simulink model "RCAM_Simulation"  (R2020a)
settings: Solver=VariableStepAuto  StartTime=0.0  StopTime=TF  RelTol=1e-3
InitFcn:
  | %Initialize constants for the RCAM simulation
  | clear; clc; close all
  | 
  | %% Define Constants
  | 
  | % Initially airplane going 165 knots at pitch of 5.73 degrees
  | x0 = [95;
  |       0;
  |       0;
  |       0;
  |       0;
  |       0;
  |       0;
  |       0.1;
  |       0];
  | 
  | x_ref = [100;
  |         0;
  |         0;
  |         0;
  |         0;
  |         0;
  |         0;
  |         0;
  |         0];
  | 
  | u = [0;
  |     -0.1;
  |     0;
  |     0.08;
  |     0.08];  % u2 initially at -5.73 degrees
  |                               % u4 and u5 at minimum initially
  | 
  | TF = 3*60;                      %sec, simulation time
  | 
  | % Saturation of Aileron Deflection, d_A
  | u1min = -25*pi/180;
  | u1max =  25*pi/180;
  | 
  | % Saturation of Tailplane (Horizontal Stabilizer) Deflection, d_T
  | u2min = -25*pi/180;
  | u2max =  10*pi/180;
  | 
  | % Saturation of Rudder Deflection, d_R
  | u3min = -30*pi/180;
  | u3max =  30*pi/180;
  | 
  | % Saturation of Throttle 1, d_TH1
  | u4min = 0.5*pi/180;
  | u4max =  10*pi/180;
  | 
  | % Saturation of Throttle 2, d_TH2
  | u5min = 0.5*pi/180;
  | u5max =  10*pi/180;
  | 
  | 
  | A_Linear = [-0.0446016164153414,0,0.0240349082743274,0,3.52183512710970,0,0,-9.80350406554132,0;
  | 0,-0.212333323695311,0,-3.64070000000000,0,-99.9337000000000,9.80350178873670,0,0;
  | -0.225748711836021,0,-0.818399711955672,0,96.6710635864611,0,0,0.357006987153097,0;
  | 0,-0.0335341188805878,0,-1.58352903033459,0,0.687344310697465,0,0,0;
  | -0.00295055240857513,0,-0.0389521422511313,0,-1.30090635747471,0,0,0,0;
  | 0,0.0108256600646234,0,0.0651934906310271,0,-0.650931103680959,0,0,0;
  | 0,0,0,1,0,-0.0364160847060240,0,0,0;
  | 0,0,0,0,1,0,0,0,0;
  | 0,0,0,0,0,1.00066284593029,0,0,0];
  | 
  | B_Linear = [0,-0.368697023171135,0,9.81000392264348,9.81000392264348;
  | 0,0,3.18499971085933,0,0;
  | 0,-10.1199839259439,0,0,0;
  | -1.31295051980772,0,0.503855989256257,0.0407489669716354,-0.0407489669716354;
  | 0,-4.03508162593975,0,0.392399973265370,0.392399973265370;
  | -0.0274928904316402,0,-0.564836211864184,0.780393997313998,-0.780393997313998;
  | 0,0,0,0,0;
  | 0,0,0,0,0;
  | 0,0,0,0,0];
  | 
  | [K_Linear,S_Linear,CLP] = lqr(A_Linear, B_Linear, eye(9), 0.1*eye(5));
StopFcn:
  | figure(1)
  | 
  | subplot(3,3,1)
  | plot(out.X.Time, out.X.Data(:,1))
  | title('velocity in x-axis')
  | xlabel('time, second')
  | ylabel('u, m/s')
  | 
  | subplot(3,3,2)
  | plot(out.X.Time, out.X.Data(:,2))
  | title('velocity in y-axis')
  | xlabel('time, second')
  | ylabel('v, m/s')
  | 
  | subplot(3,3,3)
  | plot(out.X.Time, out.X.Data(:,3))
  | title('velocity in z-axis')
  | xlabel('time, second')
  | ylabel('w, m/s')
  | 
  | subplot(3,3,4)
  | plot(out.X.Time, out.X.Data(:,4))
  | title('angular velocity about x-axis')
  | xlabel('time, second')
  | ylabel('p, rad/s')
  | 
  | subplot(3,3,5)
  | plot(out.X.Time, out.X.Data(:,5))
  | title('angular velocity about y-axis')
  | xlabel('time, second')
  | ylabel('q, rad/s')
  | 
  | subplot(3,3,6)
  | plot(out.X.Time, out.X.Data(:,6))
  | title('angular velocity about z-axis')
  | xlabel('time, second')
  | ylabel('r, rad/s')
  | 
  | subplot(3,3,7)
  | plot(out.X.Time, out.X.Data(:,7))
  | title('Roll Euler Angle')
  | xlabel('time, second')
  | ylabel('phi, rad')
  | 
  | subplot(3,3,8)
  | plot(out.X.Time, out.X.Data(:,8))
  | title('Pitch Euler Angle')
  | xlabel('time, second')
  | ylabel('theta, rad')
  | 
  | subplot(3,3,9)
  | plot(out.X.Time, out.X.Data(:,9))
  | title('Yaw Euler Angle')
  | xlabel('time, second')
  | ylabel('psi, rad')
  | 
  | Number = length(out.U.Time);
  | 
  | figure(2)
  | subplot(5,1,1)
  | plot(out.U.Time, out.U.Data(:,1))
  | title('Aileron Deflection')
  | xlabel('time, second')
  | ylabel('\delta_A, rad')
  | hold on
  | plot(out.U.Time, -25*pi/180*ones(Number),'r-')
  | plot(out.U.Time, 25*pi/180*ones(Number),'r-')
  | 
  | subplot(5,1,2)
  | plot(out.U.Time, out.U.Data(:,2))
  | title('Horizontal Stabilizer Deflection')
  | xlabel('time, second')
  | ylabel('\delta_S, rad')
  | hold on
  | plot(out.U.Time, -25*pi/180*ones(Number),'r-')
  | plot(out.U.Time, 10*pi/180*ones(Number),'r-')
  | 
  | subplot(5,1,3)
  | plot(out.U.Time, out.U.Data(:,3))
  | title('Rudder Deflection')
  | xlabel('time, second')
  | ylabel('\delta_R, rad')
  | hold on
  | plot(out.U.Time, -30*pi/180*ones(Number),'r-')
  | plot(out.U.Time, 30*pi/180*ones(Number),'r-')
  | 
  | subplot(5,1,4)
  | plot(out.U.Time, out.U.Data(:,4))
  | title('Throttle 1')
  | xlabel('time, second')
  | ylabel('\delta_th1, rad')
  | hold on
  | plot(out.U.Time, -0.5*pi/180*ones(Number),'r-')
  | plot(out.U.Time, 10*pi/180*ones(Number),'r-')
  | 
  | subplot(5,1,5)
  | plot(out.U.Time, out.U.Data(:,5))
  | title('Throttle 2')
  | xlabel('time, second')
  | ylabel('\delta_th2, rad')
  | hold on
  | plot(out.U.Time, -0.5*pi/180*ones(Number),'r-')
  | plot(out.U.Time, 10*pi/180*ones(Number),'r-')
values from neighbouring files (symbols this model uses):
  out = sim('RCAM_Simulation.slx')    [Starting_Simulation.m]
undefined symbols (not defined in the file or in its folder): K_Linear, RCAM_model
libraries: aerolibutil x2, vrlib x1
settings Model: Creator=Edward Han  LastModifiedBy=Edward Han

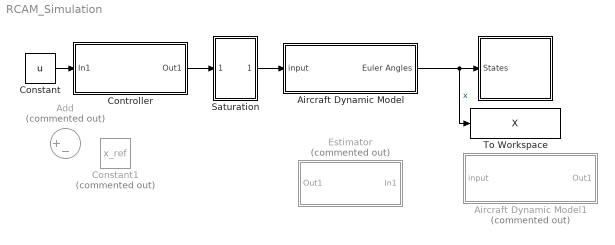
== system RCAM_Simulation ==
  " " : Subsystem
  Add : Sum  Commented=on  Inputs=|+-
  Aircraft Dynamic Model : Subsystem
  Aircraft Dynamic Model1 : Subsystem  Commented=on
  Constant : Constant  Value=u
  Constant1 : Constant  Commented=on  Value=x_ref
  Controller : Subsystem
  Estimator : Subsystem  Commented=on
  Saturation : Subsystem
  To Workspace : ToWorkspace  VariableName=X  SaveFormat=Timeseries  SampleTime=-1
  wires:
  Aircraft Dynamic Model/1(Euler Angles) -> " "/1(States), To Workspace/1  "x"
  Saturation/1(input) -> Aircraft Dynamic Model/1(input)
  Constant/1 -> Controller/1(In1)
  Controller/1(Out1) -> Saturation/1(In1)

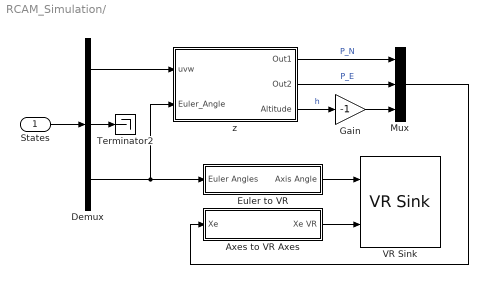
== system RCAM_Simulation/  ==
  States : Inport
  Axes to VR Axes : Subsystem
  Demux : Demux  Outputs=[3,3,3]
  Euler to VR : Subsystem
  Gain : Gain  Gain=-1
  Mux : Mux  Inputs=3
  Terminator2 : Terminator
  VR Sink : vrlib/VR Sink  InstantiateOnLoad=on  SampleTime=0.1  ViewEnable=on  RemoteChange=off  RemoteView=off  FieldsWritten=HL20.rotation.4.1.1.double#HL20.translation.3.1.1.double  WorldFileName=aeroblk_HL20.wrl  WorldDescription=aeroblk_HL20  AutoView=on  VideoDimensions=[]  AllowVariableSize=off
  z : Subsystem
  wires:
  Axes to VR Axes/1(Xe VR) -> VR Sink/2
  Euler to VR/1(Axis Angle) -> VR Sink/1
  Mux/1 -> Axes to VR Axes/1(Xe)
  States/1 -> Demux/1
  Demux/3 -> z/2(Euler_Angle), Euler to VR/1(Euler Angles)
  Demux/1 -> z/1(uvw)
  Demux/2 -> Terminator2/1
  z/3(Altitude) -> Gain/1  "h"
  z/1(Out1) -> Mux/1  "P_N"
  z/2(Out2) -> Mux/2  "P_E"
  Gain/1 -> Mux/3

== system RCAM_Simulation/Aircraft Dynamic Model ==
  input : Inport
  Integrator : Integrator  InitialCondition=x0
  Interpreted MATLAB Function : MATLABFcn  MATLABFcn=RCAM_model(u(1:9),u(10:14))
  Mux : Mux  Inputs=2
  To Workspace1 : ToWorkspace  VariableName=U  SaveFormat=Timeseries  SampleTime=-1
  Euler Angles : Outport
  wires:
  Integrator/1 -> Euler Angles/1, Mux/1
  Interpreted MATLAB Function/1 -> Integrator/1  "XDOT(9x1)"
  input/1 -> To Workspace1/1, Mux/2
  Mux/1 -> Interpreted MATLAB Function/1  "x_and_u"

== system RCAM_Simulation/Aircraft Dynamic Model1 ==
  input : Inport
  State-Space : StateSpace  A=A_Linear  B=B_Linear  C=eye(9)  D=zeros(9,5)  InitialCondition=x0
  To Workspace1 : ToWorkspace  VariableName=U  SaveFormat=Timeseries  SampleTime=-1
  Out1 : Outport
  wires:
  input/1 -> To Workspace1/1, State-Space/1
  State-Space/1 -> Out1/1

== system RCAM_Simulation/Controller ==
  In1 : Inport
  Gain : Gain  Commented=on  Gain=K_Linear  Multiplication=Matrix(K*u)
  PID : Subsystem  Commented=on
  Out1 : Outport
  wires:
  In1/1 -> Out1/1

== system RCAM_Simulation/Estimator ==
  In1 : Inport
  Out1 : Outport
  wires:
  In1/1 -> Out1/1

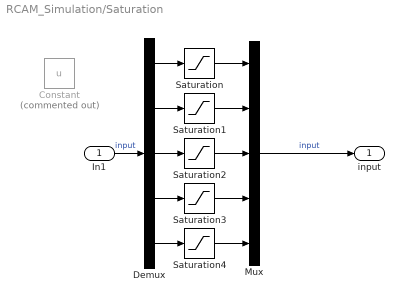
== system RCAM_Simulation/Saturation ==
  In1 : Inport
  Constant : Constant  Commented=on  Value=u
  Demux : Demux  Outputs=5
  Mux : Mux  Inputs=5
  Saturation : Saturate  UpperLimit=u1max  LowerLimit=u1min
  Saturation1 : Saturate  UpperLimit=u2max  LowerLimit=u2min
  Saturation2 : Saturate  UpperLimit=u3max  LowerLimit=u3min
  Saturation3 : Saturate  UpperLimit=u4max  LowerLimit=u4min
  Saturation4 : Saturate  UpperLimit=u5max  LowerLimit=u5min
  input : Outport
  wires:
  In1/1 -> Demux/1  "input"
  Saturation4/1 -> Mux/5
  Saturation3/1 -> Mux/4
  Demux/3 -> Saturation2/1
  Demux/1 -> Saturation/1
  Demux/2 -> Saturation1/1
  Saturation2/1 -> Mux/3
  Demux/4 -> Saturation3/1
  Demux/5 -> Saturation4/1
  Saturation/1 -> Mux/1
  Mux/1 -> input/1  "input"
  Saturation1/1 -> Mux/2

== system RCAM_Simulation/ /Axes to VR Axes ==
  Xe : Inport
  Concatenate : Concatenate  NumInputs=3
  Demux : Demux  Outputs=3
      settings: DisplayOption=none
  rad-->deg : Gain  Gain=-1  SaturateOnIntegerOverflow=on  OutDataTypeStr=Inherit: Same as input  ParamDataTypeStr=Inherit: Same as input
  rad-->deg1 : Gain  Gain=-1  SaturateOnIntegerOverflow=on  OutDataTypeStr=Inherit: Same as input  ParamDataTypeStr=Inherit: Same as input
  Xe VR : Outport  VectorParamsAs1DForOutWhenUnconnected=off
  wires:
  Xe/1 -> Demux/1
  Demux/1 -> Concatenate/1
  Demux/2 -> rad-->deg/1
  Demux/3 -> rad-->deg1/1
  Concatenate/1 -> Xe VR/1
  rad-->deg1/1 -> Concatenate/2
  rad-->deg/1 -> Concatenate/3

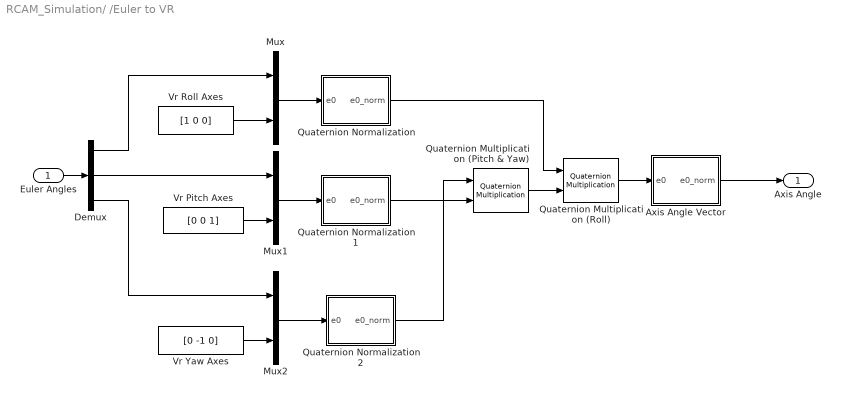
== system RCAM_Simulation/ /Euler to VR ==
  Euler Angles : Inport
  Axis Angle Vector : Subsystem
  Demux : Demux  Outputs=3
      settings: DisplayOption=none
  Mux : Mux  Inputs=2
  Mux1 : Mux  Inputs=2
  Mux2 : Mux  Inputs=2
  Quaternion Multiplication (Pitch & Yaw) : aerolibutil/Quaternion Multiplication
  Quaternion Multiplication (Roll) : aerolibutil/Quaternion Multiplication
  Quaternion Normalization : Subsystem
  Quaternion Normalization1 : Subsystem
  Quaternion Normalization2 : Subsystem
  Vr Pitch Axes : Constant  Value=[0 0 1]
  Vr Roll Axes : Constant  Value=[1 0 0]
  Vr Yaw Axes : Constant  Value=[0 -1 0]
  Axis Angle : Outport  VectorParamsAs1DForOutWhenUnconnected=off
  wires:
  Quaternion Multiplication (Roll)/1 -> Axis Angle Vector/1(e0)
  Quaternion Multiplication (Pitch & Yaw)/1 -> Quaternion Multiplication (Roll)/2
  Axis Angle Vector/1(e0_norm) -> Axis Angle/1
  Quaternion Normalization/1(e0_norm) -> Quaternion Multiplication (Roll)/1
  Quaternion Normalization2/1(e0_norm) -> Quaternion Multiplication (Pitch & Yaw)/1
  Quaternion Normalization1/1(e0_norm) -> Quaternion Multiplication (Pitch & Yaw)/2
  Mux2/1 -> Quaternion Normalization2/1(e0)
  Mux1/1 -> Quaternion Normalization1/1(e0)
  Mux/1 -> Quaternion Normalization/1(e0)
  Demux/3 -> Mux2/1
  Vr Yaw Axes/1 -> Mux2/2
  Demux/2 -> Mux1/1
  Vr Pitch Axes/1 -> Mux1/2
  Demux/1 -> Mux/1
  Vr Roll Axes/1 -> Mux/2
  Euler Angles/1 -> Demux/1

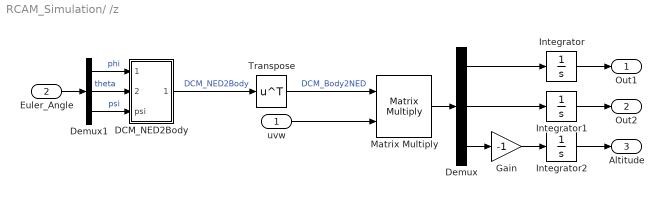
== system RCAM_Simulation/ /z ==
  uvw : Inport
  Euler_Angle : Inport  Port=2
  DCM_NED2Body : Subsystem
  Demux : Demux  Outputs=3
  Demux1 : Demux  Outputs=3
  Gain : Gain  Gain=-1
  Integrator : Integrator
  Integrator1 : Integrator
  Integrator2 : Integrator
  Matrix Multiply : Product  Multiplication=Matrix(*)
  Transpose : Math  Operator=transpose  SaturateOnIntegerOverflow=on
  Out1 : Outport
  Out2 : Outport  Port=2
  Altitude : Outport  Port=3
  wires:
  Demux1/3 -> DCM_NED2Body/3(psi)  "psi"
  Euler_Angle/1 -> Demux1/1
  Demux1/2 -> DCM_NED2Body/2(theta)  "theta"
  Demux1/1 -> DCM_NED2Body/1(phi)  "phi"
  DCM_NED2Body/1(Out3) -> Transpose/1  "DCM_NED2Body"
  Transpose/1 -> Matrix Multiply/1  "DCM_Body2NED"
  uvw/1 -> Matrix Multiply/2
  Matrix Multiply/1 -> Demux/1
  Demux/1 -> Integrator/1
  Demux/3 -> Gain/1
  Integrator/1 -> Out1/1
  Demux/2 -> Integrator1/1
  Integrator1/1 -> Out2/1
  Gain/1 -> Integrator2/1
  Integrator2/1 -> Altitude/1

== system RCAM_Simulation/Controller/PID ==
  In1 : Inport
  Add : Sum
  Demux : Demux  Outputs=[3,3,3]
  Subsystem : Subsystem
  Subsystem1 : Subsystem
  Out1 : Outport
  wires:
  In1/1 -> Demux/1
  Demux/3 -> Subsystem/2(e_att)  "e_att"
  Demux/1 -> Subsystem1/1(e_uvw)  "e_uvw"
  Subsystem/1(Out1) -> Add/2
  Demux/2 -> Subsystem/1(ed_att)  "ed_att"
  Subsystem1/1(Out1) -> Add/1
  Add/1 -> Out1/1

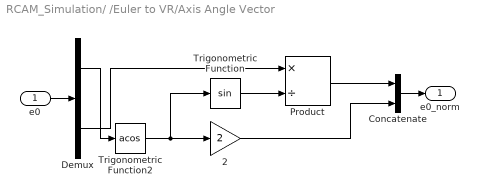
== system RCAM_Simulation/ /Euler to VR/Axis Angle Vector ==
  e0 : Inport
  2 : Gain  Gain=2  SaturateOnIntegerOverflow=on  OutDataTypeStr=Inherit: Same as input  ParamDataTypeStr=Inherit: Same as input
  Concatenate : Concatenate
  Demux : Demux  Outputs=[1 3 ]
      settings: DisplayOption=none
  Product : Product  Inputs=*/  InputSameDT=on  SaturateOnIntegerOverflow=on  OutDataTypeStr=Inherit: Same as first input
  Trigonometric Function : Trigonometry
  Trigonometric Function2 : Trigonometry  Operator=acos
  e0_norm : Outport  VectorParamsAs1DForOutWhenUnconnected=off
  wires:
  Demux/1 -> Trigonometric Function2/1
  Demux/2 -> Product/1
  Concatenate/1 -> e0_norm/1
  Product/1 -> Concatenate/1
  2/1 -> Concatenate/2
  Trigonometric Function/1 -> Product/2
  Trigonometric Function2/1 -> Trigonometric Function/1, 2/1
  e0/1 -> Demux/1

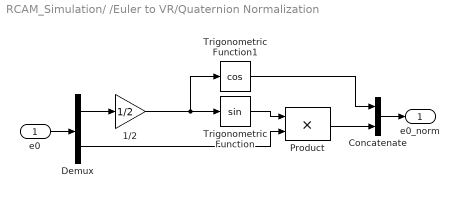
== system RCAM_Simulation/ /Euler to VR/Quaternion Normalization ==
  e0 : Inport
  1/2 : Gain  Gain=1/2  SaturateOnIntegerOverflow=on  OutDataTypeStr=Inherit: Same as input  ParamDataTypeStr=Inherit: Same as input
  Concatenate : Concatenate
  Demux : Demux  Outputs=[1 3]
      settings: DisplayOption=none
  Product : Product  InputSameDT=on  SaturateOnIntegerOverflow=on  OutDataTypeStr=Inherit: Same as first input
  Trigonometric Function : Trigonometry
  Trigonometric Function1 : Trigonometry  Operator=cos
  e0_norm : Outport  VectorParamsAs1DForOutWhenUnconnected=off
  wires:
  Trigonometric Function1/1 -> Concatenate/1
  Demux/2 -> Product/2
  Demux/1 -> 1/2/1
  Concatenate/1 -> e0_norm/1
  Product/1 -> Concatenate/2
  Trigonometric Function/1 -> Product/1
  1/2/1 -> Trigonometric Function1/1, Trigonometric Function/1
  e0/1 -> Demux/1

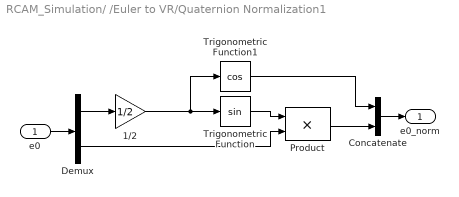
== system RCAM_Simulation/ /Euler to VR/Quaternion Normalization1 ==
  e0 : Inport
  1/2 : Gain  Gain=1/2  SaturateOnIntegerOverflow=on  OutDataTypeStr=Inherit: Same as input  ParamDataTypeStr=Inherit: Same as input
  Concatenate : Concatenate
  Demux : Demux  Outputs=[1 3]
      settings: DisplayOption=none
  Product : Product  InputSameDT=on  SaturateOnIntegerOverflow=on  OutDataTypeStr=Inherit: Same as first input
  Trigonometric Function : Trigonometry
  Trigonometric Function1 : Trigonometry  Operator=cos
  e0_norm : Outport  VectorParamsAs1DForOutWhenUnconnected=off
  wires:
  e0/1 -> Demux/1
  1/2/1 -> Trigonometric Function/1, Trigonometric Function1/1
  Trigonometric Function/1 -> Product/1
  Product/1 -> Concatenate/2
  Concatenate/1 -> e0_norm/1
  Demux/1 -> 1/2/1
  Demux/2 -> Product/2
  Trigonometric Function1/1 -> Concatenate/1

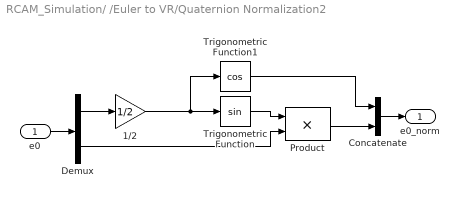
== system RCAM_Simulation/ /Euler to VR/Quaternion Normalization2 ==
  e0 : Inport
  1/2 : Gain  Gain=1/2  SaturateOnIntegerOverflow=on  OutDataTypeStr=Inherit: Same as input  ParamDataTypeStr=Inherit: Same as input
  Concatenate : Concatenate
  Demux : Demux  Outputs=[1 3]
      settings: DisplayOption=none
  Product : Product  InputSameDT=on  SaturateOnIntegerOverflow=on  OutDataTypeStr=Inherit: Same as first input
  Trigonometric Function : Trigonometry
  Trigonometric Function1 : Trigonometry  Operator=cos
  e0_norm : Outport  VectorParamsAs1DForOutWhenUnconnected=off
  wires:
  Trigonometric Function1/1 -> Concatenate/1
  Demux/2 -> Product/2
  Demux/1 -> 1/2/1
  Concatenate/1 -> e0_norm/1
  Product/1 -> Concatenate/2
  Trigonometric Function/1 -> Product/1
  1/2/1 -> Trigonometric Function1/1, Trigonometric Function/1
  e0/1 -> Demux/1

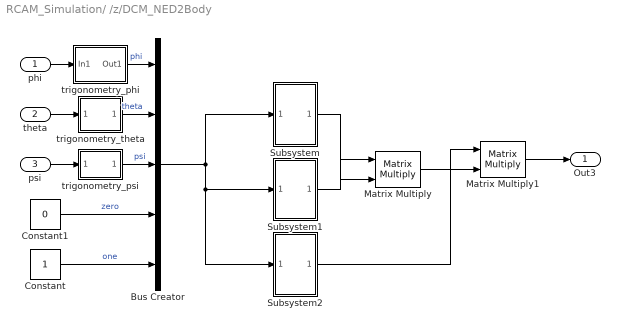
== system RCAM_Simulation/ /z/DCM_NED2Body ==
  phi : Inport
  theta : Inport  Port=2
  psi : Inport  Port=3
  Bus Creator : BusCreator  Inputs=5
  Constant : Constant
  Constant1 : Constant  Value=0
  Matrix Multiply : Product  Multiplication=Matrix(*)
  Matrix Multiply1 : Product  Multiplication=Matrix(*)
  Subsystem : Subsystem
  Subsystem1 : Subsystem
  Subsystem2 : Subsystem
  trigonometry_phi : Subsystem
  trigonometry_psi : Subsystem
  trigonometry_theta : Subsystem
  Out3 : Outport
  wires:
  Bus Creator/1 -> Subsystem2/1(In2), Subsystem1/1(In1), Subsystem/1(In1)
  phi/1 -> trigonometry_phi/1(In1)
  theta/1 -> trigonometry_theta/1(In1)
  trigonometry_phi/1(Out1) -> Bus Creator/1  "phi"
  trigonometry_theta/1(Out2) -> Bus Creator/2  "theta"
  psi/1 -> trigonometry_psi/1(In1)
  trigonometry_psi/1(Out2) -> Bus Creator/3  "psi"
  Matrix Multiply/1 -> Matrix Multiply1/2
  Matrix Multiply1/1 -> Out3/1
  Subsystem/1(Out1) -> Matrix Multiply/2
  Subsystem1/1(Out1) -> Matrix Multiply/1
  Subsystem2/1(Out1) -> Matrix Multiply1/1
  Constant1/1 -> Bus Creator/4  "zero"
  Constant/1 -> Bus Creator/5  "one"

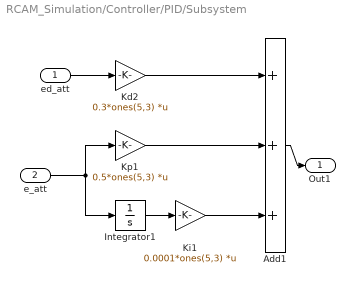
== system RCAM_Simulation/Controller/PID/Subsystem ==
  ed_att : Inport
  e_att : Inport  Port=2
  Add1 : Sum  Inputs=+++
  Integrator1 : Integrator
  Kd2 : Gain  Gain=0.3*ones(5,3)  Multiplication=Matrix(K*u)
  Ki1 : Gain  Gain=0.0001*ones(5,3)  Multiplication=Matrix(K*u)
  Kp1 : Gain  Gain=0.5*ones(5,3)  Multiplication=Matrix(K*u)
  Out1 : Outport
  wires:
  Kp1/1 -> Add1/2
  Add1/1 -> Out1/1
  Integrator1/1 -> Ki1/1
  e_att/1 -> Kp1/1, Integrator1/1
  Kd2/1 -> Add1/1
  ed_att/1 -> Kd2/1
  Ki1/1 -> Add1/3

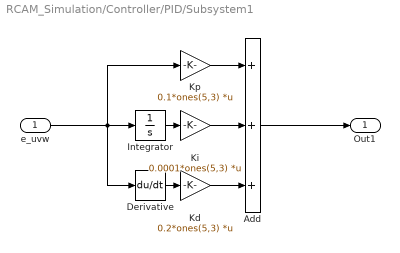
== system RCAM_Simulation/Controller/PID/Subsystem1 ==
  e_uvw : Inport
  Add : Sum  Inputs=+++
  Derivative : Derivative
  Integrator : Integrator
  Kd : Gain  Gain=0.2*ones(5,3)  Multiplication=Matrix(K*u)
  Ki : Gain  Gain=0.0001*ones(5,3)  Multiplication=Matrix(K*u)
  Kp : Gain  Gain=0.1*ones(5,3)  Multiplication=Matrix(K*u)
  Out1 : Outport
  wires:
  Ki/1 -> Add/2
  e_uvw/1 -> Derivative/1, Integrator/1, Kp/1
  Kp/1 -> Add/1
  Kd/1 -> Add/3
  Add/1 -> Out1/1
  Derivative/1 -> Kd/1
  Integrator/1 -> Ki/1

== system RCAM_Simulation/ /z/DCM_NED2Body/Subsystem ==
  In1 : Inport
  Bus Selector1 : BusSelector  OutputSignals=phi.-sphi,phi.cphi,zero  OutputAsBus=on
  Bus Selector3 : BusSelector  OutputSignals=phi.cphi,phi.sphi,zero  OutputAsBus=on
  Constant2 : Constant  Value=0
  Constant3 : Constant
  Matrix Concatenate : Concatenate  NumInputs=3  Mode=Multidimensional array  ConcatenateDimension=2
  Mux : Mux  Inputs=3
  Out1 : Outport
  wires:
  Mux/1 -> Matrix Concatenate/3
  Bus Selector3/1 -> Matrix Concatenate/1
  Bus Selector1/1 -> Matrix Concatenate/2
  Matrix Concatenate/1 -> Out1/1
  Constant3/1 -> Mux/3  "one"
  Constant2/1 -> Mux/1, Mux/2  "zero"
  In1/1 -> Bus Selector1/1, Bus Selector3/1

== system RCAM_Simulation/ /z/DCM_NED2Body/Subsystem1 ==
  In1 : Inport
  Bus Selector : BusSelector  OutputSignals=theta.ctheta,zero,theta.-stheta  OutputAsBus=on
  Bus Selector6 : BusSelector  OutputSignals=theta.stheta,zero,theta.ctheta  OutputAsBus=on
  Constant2 : Constant  Value=0
  Constant3 : Constant
  Matrix Concatenate1 : Concatenate  NumInputs=3  Mode=Multidimensional array  ConcatenateDimension=2
  Mux : Mux  Inputs=3
  Out1 : Outport
  wires:
  Bus Selector6/1 -> Matrix Concatenate1/3
  Bus Selector/1 -> Matrix Concatenate1/1
  In1/1 -> Bus Selector/1, Bus Selector6/1
  Matrix Concatenate1/1 -> Out1/1
  Constant2/1 -> Mux/3, Mux/1  "zero"
  Constant3/1 -> Mux/2  "one"
  Mux/1 -> Matrix Concatenate1/2

== system RCAM_Simulation/ /z/DCM_NED2Body/Subsystem2 ==
  In2 : Inport
  Bus Selector7 : BusSelector  OutputSignals=zero,psi.cpsi,psi.spsi  OutputAsBus=on
  Bus Selector8 : BusSelector  OutputSignals=zero,theta.-stheta,theta.ctheta  OutputAsBus=on
  Constant2 : Constant  Value=0
  Constant3 : Constant
  Matrix Concatenate2 : Concatenate  NumInputs=3  Mode=Multidimensional array  ConcatenateDimension=2
  Mux : Mux  Inputs=3
  Out1 : Outport
  wires:
  Matrix Concatenate2/1 -> Out1/1
  Bus Selector8/1 -> Matrix Concatenate2/3
  In2/1 -> Bus Selector7/1, Bus Selector8/1
  Bus Selector7/1 -> Matrix Concatenate2/2
  Mux/1 -> Matrix Concatenate2/1
  Constant3/1 -> Mux/1  "one"
  Constant2/1 -> Mux/2, Mux/3  "zero"

== system RCAM_Simulation/ /z/DCM_NED2Body/trigonometry_phi ==
  In1 : Inport
  Bus Creator : BusCreator  Inputs=4
  Gain : Gain  Gain=-1
  Gain1 : Gain  Gain=-1
  Trigonometric Function : Trigonometry
  Trigonometric Function1 : Trigonometry  Operator=cos
  Out1 : Outport
  wires:
  Trigonometric Function1/1 -> Bus Creator/1, Gain/1  "cphi"
  In1/1 -> Trigonometric Function/1, Trigonometric Function1/1
  Gain1/1 -> Bus Creator/4  "-sphi"
  Gain/1 -> Bus Creator/2  "-cphi"
  Trigonometric Function/1 -> Bus Creator/3, Gain1/1  "sphi"
  Bus Creator/1 -> Out1/1

== system RCAM_Simulation/ /z/DCM_NED2Body/trigonometry_psi ==
  In1 : Inport
  Bus Creator : BusCreator  Inputs=4
  Gain2 : Gain  Gain=-1
  Gain5 : Gain  Gain=-1
  Trigonometric Function4 : Trigonometry  Operator=cos
  Trigonometric Function5 : Trigonometry
  Out2 : Outport
  wires:
  In1/1 -> Trigonometric Function5/1, Trigonometric Function4/1
  Trigonometric Function5/1 -> Gain5/1, Bus Creator/3  "spsi"
  Trigonometric Function4/1 -> Gain2/1, Bus Creator/1  "cpsi"
  Gain5/1 -> Bus Creator/4  "-spsi"
  Gain2/1 -> Bus Creator/2  "-cpsi"
  Bus Creator/1 -> Out2/1

== system RCAM_Simulation/ /z/DCM_NED2Body/trigonometry_theta ==
  In1 : Inport
  Bus Creator : BusCreator  Inputs=4
  Gain3 : Gain  Gain=-1
  Gain4 : Gain  Gain=-1
  Trigonometric Function2 : Trigonometry  Operator=cos
  Trigonometric Function3 : Trigonometry
  Out2 : Outport
  wires:
  In1/1 -> Trigonometric Function3/1, Trigonometric Function2/1
  Trigonometric Function3/1 -> Bus Creator/3, Gain4/1  "stheta"
  Trigonometric Function2/1 -> Gain3/1, Bus Creator/1  "ctheta"
  Gain4/1 -> Bus Creator/4  "-stheta"
  Gain3/1 -> Bus Creator/2  "-ctheta"
  Bus Creator/1 -> Out2/1
